simulink model "Verification_Component_Primitive"  (R2012b)
settings: Solver=FixedStepDiscrete  StartTime=0.0  StopTime=10.0  FixedStep=0.1  RelTol=1e-3
libraries: sldvlib x15
settings Model: Creator=Kerianne  LastModifiedBy=Kerianne
settings DataIOCC: SaveFormat=Structure
settings OptimizationCC: InlineParams=on

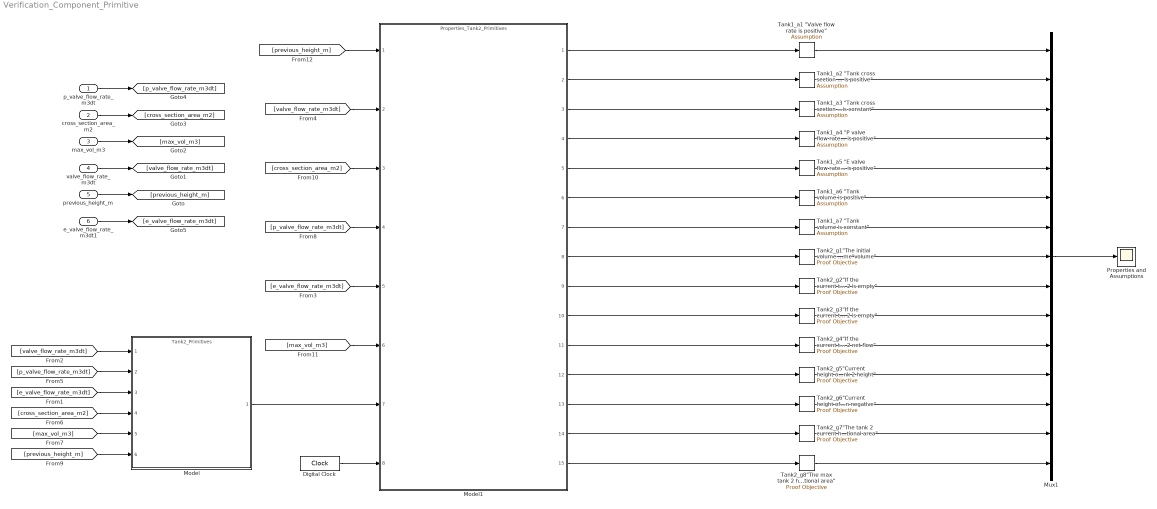
== system Verification_Component_Primitive ==
  p_valve_flow_rate_m3dt : Inport  OutDataTypeStr=double
  cross_section_area_m2 : Inport  Port=2  OutDataTypeStr=double
  max_vol_m3 : Inport  Port=3  OutDataTypeStr=double
  valve_flow_rate_m3dt : Inport  Port=4  OutDataTypeStr=double
  previous_height_m : Inport  Port=5  OutDataTypeStr=double
  e_valve_flow_rate_m3dt1 : Inport  Port=6  OutDataTypeStr=double
  Digital Clock : DigitalClock  SampleTime=0.1
  Model : ModelReference  ModelNameDialog=Tank2_Primitives  SimulationMode=Normal  ModelReferenceVersion=1.30  CopyOfModelName=Tank2_Primitives  DefaultDataLogging=on
  Model1 : ModelReference  ModelNameDialog=Properties_Tank2_Primitives  SimulationMode=Normal  ModelReferenceVersion=1.23  CopyOfModelName=Properties_Tank2_Primitives  DefaultDataLogging=on
  Mux1 : Mux  Inputs=15
  Properties and Assumptions : Scope
      settings: ShowLegends=on
  "Tank1_a1 \"Valve flow rate is positive\"" : sldvlib/Objectives and Constraints/Assumption  enabled=on  customAVTBlockType=Assumption  intervals=true  initial=off  dispValues=on  outEnabled=on
      settings: AttributesFormatString=%<intervals>
  "Tank1_a2 \"Tank cross section area is positive\"" : sldvlib/Objectives and Constraints/Assumption  enabled=on  customAVTBlockType=Assumption  intervals=true  initial=off  dispValues=on  outEnabled=on
      settings: AttributesFormatString=%<intervals>
  "Tank1_a3 \"Tank cross section area is constant\"" : sldvlib/Objectives and Constraints/Assumption  enabled=on  customAVTBlockType=Assumption  intervals=true  initial=off  dispValues=on  outEnabled=on
      settings: AttributesFormatString=%<intervals>
  "Tank1_a4 \"P valve flow rate is positive\"" : sldvlib/Objectives and Constraints/Assumption  enabled=on  customAVTBlockType=Assumption  intervals=true  initial=off  dispValues=on  outEnabled=on
      settings: AttributesFormatString=%<intervals>
  "Tank1_a5 \"E valve flow rate is positive\"" : sldvlib/Objectives and Constraints/Assumption  enabled=on  customAVTBlockType=Assumption  intervals=true  initial=off  dispValues=on  outEnabled=on
      settings: AttributesFormatString=%<intervals>
  "Tank1_a6 \"Tank volume is positive\"" : sldvlib/Objectives and Constraints/Assumption  enabled=on  customAVTBlockType=Assumption  intervals=true  initial=off  dispValues=on  outEnabled=on
      settings: AttributesFormatString=%<intervals>
  "Tank1_a7 \"Tank volume is constant\"" : sldvlib/Objectives and Constraints/Assumption  enabled=on  customAVTBlockType=Assumption  intervals=true  initial=off  dispValues=on  outEnabled=on
      settings: AttributesFormatString=%<intervals>
  "Tank2_g1\"The initial volume of tank 2 should be equivalent to the specified initial tank 2 volume\"volume\" " : sldvlib/Objectives and Constraints/Proof Objective  enabled=on  customAVTBlockType=Proof Objective  intervals=true  dispValues=on  outEnabled=on  enableStopSim=off
      settings: AttributesFormatString=%<intervals>
  "Tank2_g2\"If the current tank 2 volume plus the tank 2 net flow is less than the tank 2 minimum volume then tank 2 is empty\" " : sldvlib/Objectives and Constraints/Proof Objective  enabled=on  customAVTBlockType=Proof Objective  intervals=true  dispValues=on  outEnabled=on  enableStopSim=off
      settings: AttributesFormatString=%<intervals>
  "Tank2_g3\"If the current tank 2 volume plus the tank 2 net flow is less than the tank 2 minimum volume then tank 2 is empty\"" : sldvlib/Objectives and Constraints/Proof Objective  enabled=on  customAVTBlockType=Proof Objective  intervals=true  dispValues=on  outEnabled=on  enableStopSim=off
      settings: AttributesFormatString=%<intervals>
  "Tank2_g4\"If the current tank 2 volume plus the tank 2 net flow is greater than empty and less than the tank 2 maximum volume then the tank 2 volume changes by the tank 2 net flow\"" : sldvlib/Objectives and Constraints/Proof Objective  enabled=on  customAVTBlockType=Proof Objective  intervals=true  dispValues=on  outEnabled=on  enableStopSim=off
      settings: AttributesFormatString=%<intervals>
  "Tank2_g5\"Current height of tank 2 is equal or less than the max tank 2 height\"" : sldvlib/Objectives and Constraints/Proof Objective  enabled=on  customAVTBlockType=Proof Objective  intervals=true  dispValues=on  outEnabled=on  enableStopSim=off
      settings: AttributesFormatString=%<intervals>
  "Tank2_g6\"Current height of tank 2 is non negative\"" : sldvlib/Objectives and Constraints/Proof Objective  enabled=on  customAVTBlockType=Proof Objective  intervals=true  dispValues=on  outEnabled=on  enableStopSim=off
      settings: AttributesFormatString=%<intervals>
  "Tank2_g7\"The tank 2 current height is equal to the tank 2 current volume divided by the tank 2 cross sectional area\" " : sldvlib/Objectives and Constraints/Proof Objective  enabled=on  customAVTBlockType=Proof Objective  intervals=true  dispValues=on  outEnabled=on  enableStopSim=off
      settings: AttributesFormatString=%<intervals>
  "Tank2_g8\"The max tank 2 height is equal to the max tank 2 volume divided by tank 2 cross sectional area\"" : sldvlib/Objectives and Constraints/Proof Objective  enabled=on  customAVTBlockType=Proof Objective  intervals=true  dispValues=on  outEnabled=on  enableStopSim=off
      settings: AttributesFormatString=%<intervals>
  wires:
  Model/1 -> Model1/7
  Mux1/1 -> Properties and Assumptions/1
  previous_height_m/1 -> [previous_height_m]
  valve_flow_rate_m3dt/1 -> [valve_flow_rate_m3dt]
  max_vol_m3/1 -> [max_vol_m3]
  p_valve_flow_rate_m3dt/1 -> [p_valve_flow_rate_m3dt]
  cross_section_area_m2/1 -> [cross_section_area_m2]
  Digital Clock/1 -> Model1/8
  e_valve_flow_rate_m3dt1/1 -> [e_valve_flow_rate_m3dt]
  [valve_flow_rate_m3dt] -> Model/1
  [p_valve_flow_rate_m3dt] -> Model/2
  [e_valve_flow_rate_m3dt] -> Model/3
  [cross_section_area_m2] -> Model/4
  [max_vol_m3] -> Model/5
  [previous_height_m] -> Model/6
  [previous_height_m] -> Model1/1
  [valve_flow_rate_m3dt] -> Model1/2
  [cross_section_area_m2] -> Model1/3
  [p_valve_flow_rate_m3dt] -> Model1/4
  [e_valve_flow_rate_m3dt] -> Model1/5
  [max_vol_m3] -> Model1/6
  Model1/7 -> "Tank1_a7 \"Tank volume is constant\""/1
  Model1/6 -> "Tank1_a6 \"Tank volume is positive\""/1
  Model1/5 -> "Tank1_a5 \"E valve flow rate is positive\""/1
  Model1/4 -> "Tank1_a4 \"P valve flow rate is positive\""/1
  Model1/3 -> "Tank1_a3 \"Tank cross section area is constant\""/1
  Model1/2 -> "Tank1_a2 \"Tank cross section area is positive\""/1
  Model1/1 -> "Tank1_a1 \"Valve flow rate is positive\""/1
  "Tank1_a1 \"Valve flow rate is positive\""/1 -> Mux1/1
  "Tank1_a2 \"Tank cross section area is positive\""/1 -> Mux1/2
  "Tank1_a3 \"Tank cross section area is constant\""/1 -> Mux1/3
  "Tank1_a4 \"P valve flow rate is positive\""/1 -> Mux1/4
  "Tank1_a5 \"E valve flow rate is positive\""/1 -> Mux1/5
  "Tank1_a6 \"Tank volume is positive\""/1 -> Mux1/6
  "Tank1_a7 \"Tank volume is constant\""/1 -> Mux1/7
  Model1/8 -> "Tank2_g1\"The initial volume of tank 2 should be equivalent to the specified initial tank 2 volume\"volume\" "/1
  Model1/9 -> "Tank2_g2\"If the current tank 2 volume plus the tank 2 net flow is less than the tank 2 minimum volume then tank 2 is empty\" "/1
  Model1/10 -> "Tank2_g3\"If the current tank 2 volume plus the tank 2 net flow is less than the tank 2 minimum volume then tank 2 is empty\""/1
  Model1/11 -> "Tank2_g4\"If the current tank 2 volume plus the tank 2 net flow is greater than empty and less than the tank 2 maximum volume then the tank 2 volume changes by the tank 2 net flow\""/1
  Model1/12 -> "Tank2_g5\"Current height of tank 2 is equal or less than the max tank 2 height\""/1
  Model1/13 -> "Tank2_g6\"Current height of tank 2 is non negative\""/1
  Model1/14 -> "Tank2_g7\"The tank 2 current height is equal to the tank 2 current volume divided by the tank 2 cross sectional area\" "/1
  Model1/15 -> "Tank2_g8\"The max tank 2 height is equal to the max tank 2 volume divided by tank 2 cross sectional area\""/1
  "Tank2_g1\"The initial volume of tank 2 should be equivalent to the specified initial tank 2 volume\"volume\" "/1 -> Mux1/8
  "Tank2_g2\"If the current tank 2 volume plus the tank 2 net flow is less than the tank 2 minimum volume then tank 2 is empty\" "/1 -> Mux1/9
  "Tank2_g3\"If the current tank 2 volume plus the tank 2 net flow is less than the tank 2 minimum volume then tank 2 is empty\""/1 -> Mux1/10
  "Tank2_g4\"If the current tank 2 volume plus the tank 2 net flow is greater than empty and less than the tank 2 maximum volume then the tank 2 volume changes by the tank 2 net flow\""/1 -> Mux1/11
  "Tank2_g5\"Current height of tank 2 is equal or less than the max tank 2 height\""/1 -> Mux1/12
  "Tank2_g6\"Current height of tank 2 is non negative\""/1 -> Mux1/13
  "Tank2_g7\"The tank 2 current height is equal to the tank 2 current volume divided by the tank 2 cross sectional area\" "/1 -> Mux1/14
  "Tank2_g8\"The max tank 2 height is equal to the max tank 2 volume divided by tank 2 cross sectional area\""/1 -> Mux1/15
